simulink model "ppf1"  (R2020b)
settings: Solver=VariableStepAuto  StartTime=0.0  StopTime=10.0  RelTol=1e-3
settings Model: Creator=xinxinzhang  LastModifiedBy=xinxinzhang

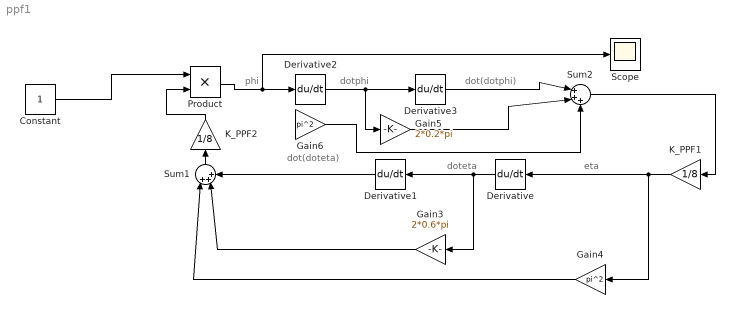
== system ppf1 ==
  note: phi
  note: dotphi
  note: dot(dotphi)
  note: eta
  note: doteta
  note: dot(doteta)
  Constant : Constant
  Derivative{,1..3} (4 alike) : Derivative
  Gain3 : Gain  Gain=2*0.6*pi
  Gain4 : Gain  Gain=pi^2
  Gain5 : Gain  Gain=2*0.2*pi
  Gain6 : Gain  Gain=pi^2
  K_PPF1 : Gain  Gain=1/8
  K_PPF2 : Gain  Gain=1/8
  Product : Product
  Scope : Scope
  Sum1 : Sum  Inputs=|+++
  Sum2 : Sum  Inputs=|+++
  wires:
  K_PPF1/1 -> Gain4/1, Derivative/1
  Derivative/1 -> Gain3/1, Derivative1/1
  Derivative1/1 -> Sum1/3
  Gain3/1 -> Sum1/2
  Gain4/1 -> Sum1/1
  Sum1/1 -> K_PPF2/1
  Derivative2/1 -> Gain5/1, Derivative3/1
  Derivative3/1 -> Sum2/1
  Gain6/1 -> Sum2/3
  Gain5/1 -> Sum2/2
  Sum2/1 -> K_PPF1/1
  Constant/1 -> Product/1
  K_PPF2/1 -> Product/2
  Product/1 -> Scope/1, Derivative2/1
